simulink model "simulink_app"  (R2015a)
settings: Solver=ode2  SolverMode=SingleTasking  StartTime=0.0  StopTime=inf  FixedStep=T_ctrl  RelTol=1e-3
undefined symbols (not defined in the file): A_l_max_x, A_l_max_y, A_z_max, B_hover_4dof, CG_0, epsilon, eta_23, g, h, h_M, Hover_eta_23, Hover_throtle_1, Hover_throtle_23, I_BAC_0, Ix, Iy, Iz, l, l_arm, m, m_0, m_M, Rotation_sign, T_ctrl, throtle_1, throtle_23, v_i0
libraries: XXCopter_Control x52, simulink x11, XXCopter x1
(part 1 of 4)
settings Model: ExtModeTrigDuration=5000  Creator=DavidTorres  LastModifiedBy=David
settings SolverCC: AutoInsertRateTranBlk=on
settings DataIOCC: LimitDataPoints=off  SaveOutput=off  SignalLogging=off  DSMLogging=off  VisualizeSimOutput=off  SaveTime=off
settings OptimizationCC: InlineParams=on  UseFloatMulNetSlope=on  UseSpecifiedMinMax=on  InlineInvariantSignals=on  EnhancedBackFolding=on  PassReuseOutputArgsAs=Individual arguments  EfficientFloat2IntCast=on  EfficientMapNaN2IntZero=off  LifeSpan=Inf  MaxStackSize=64
settings DebuggingCC: WriteAfterWriteMsg=EnableAllAsError  SaveWithParameterizedLinksMsg=none  SignalResolutionControl=TryResolveAllWithWarning  IntegerOverflowMsg=error  ParameterUnderflowMsg=error  ParameterTunabilityLossMsg=error  UniqueDataStoreMsg=error  StrictBusMsg=ErrorOnBusTreatedAsVector  NonBusSignalsTreatedAsBus=error  SFUnexpectedBacktrackingDiag=error  SFInvalidInputDataAccessInChartInitDiag=error  SFNoUnconditionalDefaultTransitionDiag=error  SFTransitionOutsideNaturalParentDiag=error  SFUnconditionalTransitionShadowingDiag=error  SFUndirectedBroadcastEventsDiag=error  SFTransitionActionBeforeConditionDiag=error  IntegerSaturationMsg=error
settings HardwareCC: ProdLargestAtomicInteger=Long  ProdLargestAtomicFloat=Double  ProdEndianess=LittleEndian  ProdHWDeviceType=ARM Compatible->ARM Cortex
settings RTWCC: SystemTargetFile=ert.tlc  GenCodeOnly=on  TemplateMakefile=ert_default_tmf  Description=Embedded Coder  Toolchain=GNU Tools for ARM Embedded Processors  BuildConfiguration=Faster Runs
settings CodeAppCC: IgnoreCustomStorageClasses=off  IgnoreTestpoints=on
settings ERTTargetCC: UtilityFuncGeneration=Shared location  ParMdlRefBuildCompliant=on  CompOptLevelCompliant=on  ConcurrentExecutionCompliant=on  IncludeMdlTerminateFcn=off  ERTFirstTimeCompliant=on  ParenthesesLevel=Minimum  ModelStepFunctionPrototypeControlCompliant=on  CPPClassGenCompliant=on  ERTCustomFileTemplate=example_file_process.tlc  PreserveIfCondition=on  ConvertIfToSwitch=on

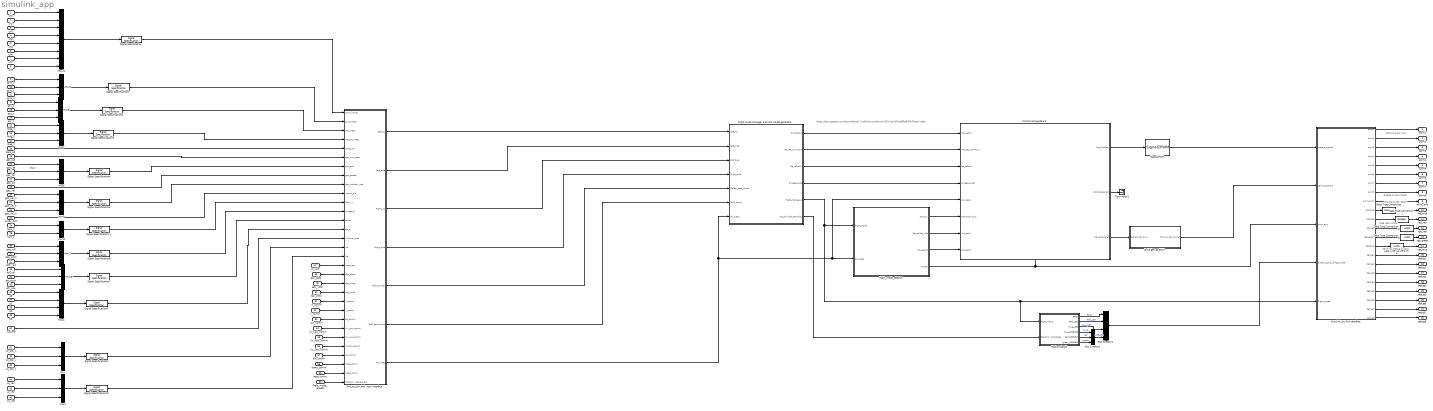
== system simulink_app ==
  note: degs!
  note: https://docs.google.com/document/d/17Lw5HdxcxpxePsmAYdCNVeyrDDt4j9EbtB6DkGHaHsY/edit
  note: Terminal Debug Output
  note: RGB LED (uint8)
  note: Standard LED (Bool)
  note: PWM Output (uS)
  note: Enable Output (Bool)
  ch1 : Inport  PortDimensions=[1,1]  SampleTime=T_ctrl
  ch2 : Inport  Port=2  PortDimensions=[1,1]  SampleTime=T_ctrl
  ch3 : Inport  Port=3  PortDimensions=[1,1]  SampleTime=T_ctrl
  ch4 : Inport  Port=4  PortDimensions=[1,1]  SampleTime=T_ctrl
  ch5 : Inport  Port=5  PortDimensions=[1,1]  SampleTime=T_ctrl
  ch6 : Inport  Port=6  PortDimensions=[1,1]  SampleTime=T_ctrl
  ch7 : Inport  Port=7  PortDimensions=[1,1]  SampleTime=T_ctrl
  ch8 : Inport  Port=8  PortDimensions=[1,1]  SampleTime=T_ctrl
  gyro_x : Inport  Port=9  PortDimensions=[1,1]  SampleTime=T_ctrl
  gyro_y : Inport  Port=10  PortDimensions=[1,1]  SampleTime=T_ctrl
  gyro_z : Inport  Port=11  PortDimensions=[1,1]  SampleTime=T_ctrl
  acc_x : Inport  Port=12  PortDimensions=[1,1]  SampleTime=T_ctrl
  acc_y : Inport  Port=13  PortDimensions=[1,1]  SampleTime=T_ctrl
  acc_z : Inport  Port=14  PortDimensions=[1,1]  SampleTime=T_ctrl
  mag_x : Inport  Port=15  PortDimensions=[1,1]  SampleTime=T_ctrl
  mag_y : Inport  Port=16  PortDimensions=[1,1]  SampleTime=T_ctrl
  mag_z : Inport  Port=17  PortDimensions=[1,1]  SampleTime=T_ctrl
  baro_alt : Inport  Port=18  PortDimensions=[1,1]  SampleTime=T_ctrl
  gps_sat : Inport  Port=19  PortDimensions=[1,1]  SampleTime=T_ctrl
  gps_lat : Inport  Port=20  PortDimensions=[1,1]  SampleTime=T_ctrl
  gps_lon : Inport  Port=21  PortDimensions=[1,1]  SampleTime=T_ctrl
  gps_alt : Inport  Port=22  PortDimensions=[1,1]  SampleTime=T_ctrl
  gps_vel : Inport  Port=23  PortDimensions=[1,1]  SampleTime=T_ctrl
  gps_vel_n : Inport  Port=24  PortDimensions=[1,1]  SampleTime=T_ctrl
  gps_vel_e : Inport  Port=25  PortDimensions=[1,1]  SampleTime=T_ctrl
  gps_vel_d : Inport  Port=26  PortDimensions=[1,1]  SampleTime=T_ctrl
  sonar_dist : Inport  Port=27  PortDimensions=[1,1]  SampleTime=T_ctrl
  flow_x : Inport  Port=28  PortDimensions=[1,1]  SampleTime=T_ctrl
  flow_y : Inport  Port=29  PortDimensions=[1,1]  SampleTime=T_ctrl
  rate_roll : Inport  Port=30  PortDimensions=[1,1]  SampleTime=T_ctrl
  rate_pitch : Inport  Port=31  PortDimensions=[1,1]  SampleTime=T_ctrl
  rate_yaw : Inport  Port=32  PortDimensions=[1,1]  SampleTime=T_ctrl
  att_roll : Inport  Port=33  PortDimensions=[1,1]  SampleTime=T_ctrl
  att_pitch : Inport  Port=34  PortDimensions=[1,1]  SampleTime=T_ctrl
  att_yaw : Inport  Port=35  PortDimensions=[1,1]  SampleTime=T_ctrl
  q0 : Inport  Port=36  PortDimensions=[1,1]  SampleTime=T_ctrl
  q1 : Inport  Port=37  PortDimensions=[1,1]  SampleTime=T_ctrl
  q2 : Inport  Port=38  PortDimensions=[1,1]  SampleTime=T_ctrl
  q3 : Inport  Port=39  PortDimensions=[1,1]  SampleTime=T_ctrl
  runtime : Inport  Port=40  PortDimensions=[1,1]  SampleTime=T_ctrl
  Lo_pos_x : Inport  Port=41  PortDimensions=[1,1]  SampleTime=T_ctrl
  Lo_pos_y : Inport  Port=42  PortDimensions=[1,1]  SampleTime=T_ctrl
  Lo_pos_z : Inport  Port=43  PortDimensions=[1,1]  SampleTime=T_ctrl
  Lo_vex : Inport  Port=44  PortDimensions=[1,1]  SampleTime=T_ctrl
  Lo_vey : Inport  Port=45  PortDimensions=[1,1]  SampleTime=T_ctrl
  Lo_vez : Inport  Port=46  PortDimensions=[1,1]  SampleTime=T_ctrl
  Lo_yaw : Inport  Port=47  PortDimensions=[1,1]  SampleTime=T_ctrl
  gps_pdop : Inport  Port=48  PortDimensions=[1,1]  SampleTime=T_ctrl
  gps_vdop : Inport  Port=49  PortDimensions=[1,1]  SampleTime=T_ctrl
  bat_volts : Inport  Port=50  PortDimensions=[1,1]  SampleTime=T_ctrl
  X_comm : Inport  Port=51  PortDimensions=[1,1]  SampleTime=T_ctrl
  Y_comm : Inport  Port=52  PortDimensions=[1,1]  SampleTime=T_ctrl
  Alt_comm : Inport  Port=53  PortDimensions=[1,1]  SampleTime=T_ctrl
  Vx_yaw_comm : Inport  Port=54  PortDimensions=[1,1]  SampleTime=T_ctrl
  Vy_yaw_comm : Inport  Port=55  PortDimensions=[1,1]  SampleTime=T_ctrl
  Vz_yaw_comm : Inport  Port=56  PortDimensions=[1,1]  SampleTime=T_ctrl
  phi_comm : Inport  Port=57  PortDimensions=[1,1]  SampleTime=T_ctrl
  theta_comm : Inport  Port=58  PortDimensions=[1,1]  SampleTime=T_ctrl
  head_comm : Inport  Port=59  PortDimensions=[1,1]  SampleTime=T_ctrl
  flight_mode_request : Inport  Port=60  PortDimensions=[1,1]  SampleTime=T_ctrl
  Build Servos PWM : Subsystem  TreatAsAtomicUnit=on
  Bus Creator1 : BusCreator
  Bus Creator2 : BusCreator  Inputs=3
  Control and guidance : Subsystem
  Data Type Conversion : DataTypeConversion  OutDataTypeStr=boolean
  Data Type Conversion1 : DataTypeConversion  OutDataTypeStr=boolean
  Data Type Conversion2 : DataTypeConversion  OutDataTypeStr=uint8
  Data Type Conversion3 : DataTypeConversion  OutDataTypeStr=uint8
  Data Type Conversion4 : DataTypeConversion  OutDataTypeStr=uint8
  Flight mode manager and commands generator : Subsystem
  Mux{,1..3,5..9} (9 alike) : Mux  Inputs=3
  Mux10 : Mux  Inputs=2
  Mux11 : Mux  Inputs=8
  Mux4 : Mux
  Px4_to_simulink input interface : Subsystem
  Signal Specification : SignalSpecification  Dimensions=[8,1]
  Signal Specification{1..7,9..10} (9 alike) : SignalSpecification  Dimensions=[3,1]
  Signal Specification11 : SignalSpecification  Dimensions=[2,1]
  Signal Specification8 : SignalSpecification  Dimensions=[4,1]
  Signal2PWM : XXCopter_Control/Signal2PWM  b=1  d=0  a=1800  c=1200
  Simulink_to_Px4 interface : Subsystem
  Status signals : Subsystem  TreatAsAtomicUnit=on
  Terminator1 : Terminator
  flight_mode_effector : Subsystem
  pwm1 : Outport  PortDimensions=[1,1]
  pwm2 : Outport  Port=2  PortDimensions=[1,1]
  pwm3 : Outport  Port=3  PortDimensions=[1,1]
  pwm4 : Outport  Port=4  PortDimensions=[1,1]
  pwm5 : Outport  Port=5  PortDimensions=[1,1]
  pwm6 : Outport  Port=6  PortDimensions=[1,1]
  pwm7 : Outport  Port=7  PortDimensions=[1,1]
  pwm8 : Outport  Port=8  PortDimensions=[1,1]
  pwm_arm : Outport  Port=9  PortDimensions=[1,1]
  led_blue : Outport  Port=10  OutDataTypeStr=boolean  PortDimensions=[1,1]
  led_red : Outport  Port=11  OutDataTypeStr=boolean  PortDimensions=[1,1]
  rgb_red : Outport  Port=12  OutDataTypeStr=uint8  PortDimensions=[1,1]
  rgb_green : Outport  Port=13  OutDataTypeStr=uint8  PortDimensions=[1,1]
  rgb_blue : Outport  Port=14  OutDataTypeStr=uint8  PortDimensions=[1,1]
  debug1 : Outport  Port=15  PortDimensions=[1,1]
  debug2 : Outport  Port=16  PortDimensions=[1,1]
  debug3 : Outport  Port=17  PortDimensions=[1,1]
  debug4 : Outport  Port=18  PortDimensions=[1,1]
  debug5 : Outport  Port=19  PortDimensions=[1,1]
  debug6 : Outport  Port=20  PortDimensions=[1,1]
  debug7 : Outport  Port=21  PortDimensions=[1,1]
  debug8 : Outport  Port=22  PortDimensions=[1,1]
  wires:
  Flight mode manager and commands generator/1(Pos_ref(m)) -> Control and guidance/1(Pos_ref(m))
  Flight mode manager and commands generator/2(Vel_ref_yaw(mps)) -> Control and guidance/2(Vel_ref_yaw(mps))
  Flight mode manager and commands generator/3(Att_ref(rad)) -> Control and guidance/3(Att_ref(rad))
  Control and guidance/1(Mot_throtles) -> Signal2PWM/1
  Control and guidance/3(Servos_angles) -> Build Servos PWM/1(signals servos in)
  Flight mode manager and commands generator/4(omega_b_ref) -> Control and guidance/4(omega_b_ref)
  flight_mode_effector/1(Act_bus) -> Control and guidance/6(activation_bus)
  flight_mode_effector/2(Controller_inits) -> Control and guidance/7(Init_cond)
  flight_mode_effector/3(CA_reconf) -> Control and guidance/8(CA_reconf)
  Flight mode manager and commands generator/6(not_allowed_transition) -> Status signals/2(Not_allowed_change)
  Status signals/1(Beep) -> Bus Creator1/1  "Beep"
  Status signals/2(Red_LED) -> Bus Creator1/2  "Red_LED"
  Status signals/3(blue_LED) -> Bus Creator1/3  "blue_LED"
  Status signals/4(blue_RGBLED) -> Bus Creator2/1  "blue"
  Status signals/5(Red_RGBLED) -> Bus Creator2/2  "red"
  Status signals/6(green_RGBLED) -> Bus Creator2/3  "green"
  Bus Creator2/1 -> Bus Creator1/4  "RGBLED"
  Simulink_to_Px4 interface/1(pwm1) -> pwm1/1
  Simulink_to_Px4 interface/2(pwm2) -> pwm2/1
  Simulink_to_Px4 interface/3(pwm3) -> pwm3/1
  Simulink_to_Px4 interface/4(pwm4) -> pwm4/1
  Simulink_to_Px4 interface/5(pwm5) -> pwm5/1
  Simulink_to_Px4 interface/6(pwm6) -> pwm6/1
  Simulink_to_Px4 interface/7(pwm7) -> pwm7/1
  Simulink_to_Px4 interface/8(pwm8) -> pwm8/1
  Simulink_to_Px4 interface/10(led_blue) -> Data Type Conversion/1
  Simulink_to_Px4 interface/11(led_red) -> Data Type Conversion1/1
  Simulink_to_Px4 interface/15(debug1) -> debug1/1
  Simulink_to_Px4 interface/17(debug3) -> debug3/1
  Simulink_to_Px4 interface/18(debug4) -> debug4/1
  Simulink_to_Px4 interface/9(pwm_arm1) -> pwm_arm/1
  Simulink_to_Px4 interface/12(rgb_red) -> Data Type Conversion2/1
  Simulink_to_Px4 interface/13(rgb_green) -> Data Type Conversion3/1
  Simulink_to_Px4 interface/14(rgb_blue) -> Data Type Conversion4/1
  Simulink_to_Px4 interface/20(debug6) -> debug6/1
  Simulink_to_Px4 interface/21(debug7) -> debug7/1
  Simulink_to_Px4 interface/22(debug8) -> debug8/1
  Simulink_to_Px4 interface/19(debug5) -> debug5/1
  flight_mode_effector/4(Armed) -> Simulink_to_Px4 interface/3(pwm_arm), Control and guidance/Enable
  Data Type Conversion/1 -> led_blue/1
  Data Type Conversion1/1 -> led_red/1
  Flight mode manager and commands generator/5(flight_mode_out) -> Simulink_to_Px4 interface/5(flight_mode), Status signals/1(flight_mode), flight_mode_effector/1(flight_mode)
  Data Type Conversion2/1 -> rgb_red/1
  Data Type Conversion3/1 -> rgb_green/1
  Data Type Conversion4/1 -> rgb_blue/1
  Control and guidance/2(Control_signals) -> Terminator1/1
  Simulink_to_Px4 interface/16(debug2) -> debug2/1
  Signal2PWM/1 -> Simulink_to_Px4 interface/1(motors_signals)
  Build Servos PWM/1(PWM_us servos out) -> Simulink_to_Px4 interface/2(servos_signals)
  Bus Creator1/1 -> Simulink_to_Px4 interface/4(extern_signal_flihgt_mode)
  Px4_to_simulink input interface/7(All_meas) -> Control and guidance/5(All_meas), flight_mode_effector/2(All_meas), Flight mode manager and commands generator/7(All_meas)
  sonar_dist/1 -> Px4_to_simulink input interface/10(usonic_alt)
  baro_alt/1 -> Px4_to_simulink input interface/5(press_alt)
  gyro_z/1 -> Mux6/3
  gyro_y/1 -> Mux6/2
  gyro_x/1 -> Mux6/1
  acc_z/1 -> Mux5/3
  acc_y/1 -> Mux5/2
  acc_x/1 -> Mux5/1
  mag_x/1 -> Mux7/1
  mag_y/1 -> Mux7/2
  mag_z/1 -> Mux7/3
  ch1/1 -> Mux11/1
  ch2/1 -> Mux11/2
  ch3/1 -> Mux11/3
  ch4/1 -> Mux11/4
  ch5/1 -> Mux11/5
  ch6/1 -> Mux11/6
  flow_y/1 -> Mux10/2
  flow_x/1 -> Mux10/1
  runtime/1 -> Px4_to_simulink input interface/15(runtime_usec)
  ch7/1 -> Mux11/7
  ch8/1 -> Mux11/8
  att_roll/1 -> Mux3/1
  att_pitch/1 -> Mux3/2
  att_yaw/1 -> Mux3/3
  q0/1 -> Mux4/1
  q1/1 -> Mux4/2
  q2/1 -> Mux4/3
  q3/1 -> Mux4/4
  rate_roll/1 -> Mux2/1
  rate_pitch/1 -> Mux2/2
  rate_yaw/1 -> Mux2/3
  gps_vel_n/1 -> Mux9/1
  gps_vel_e/1 -> Mux9/2
  gps_vel_d/1 -> Mux9/3
  gps_lat/1 -> Mux8/1
  gps_lon/1 -> Mux8/2
  gps_alt/1 -> Mux8/3
  gps_vel/1 -> Px4_to_simulink input interface/8(gps_speed)
  gps_sat/1 -> Px4_to_simulink input interface/6(gps_num_sats)
  Lo_pos_x/1 -> Mux/1
  Lo_pos_y/1 -> Mux/2
  Lo_pos_z/1 -> Mux/3
  Mux/1 -> Signal Specification9/1
  Lo_vex/1 -> Mux1/1
  Lo_vey/1 -> Mux1/2
  Lo_vez/1 -> Mux1/3
  Mux1/1 -> Signal Specification10/1
  Mux2/1 -> Signal Specification6/1
  Mux3/1 -> Signal Specification7/1
  Mux4/1 -> Signal Specification8/1
  Mux5/1 -> Signal Specification2/1
  Y_comm/1 -> Px4_to_simulink input interface/23(Y_comm)
  Alt_comm/1 -> Px4_to_simulink input interface/24(Alt_comm)
  Vx_yaw_comm/1 -> Px4_to_simulink input interface/25(Vx_yaw_comm)
  Vy_yaw_comm/1 -> Px4_to_simulink input interface/26(Vy_yaw_comm)
  theta_comm/1 -> Px4_to_simulink input interface/29(theta_comm)
  head_comm/1 -> Px4_to_simulink input interface/30(head_comm)
  flight_mode_request/1 -> Px4_to_simulink input interface/31(flight_mode_request)
  Mux6/1 -> Signal Specification1/1
  Mux8/1 -> Signal Specification4/1
  Mux7/1 -> Signal Specification3/1
  Mux11/1 -> Signal Specification/1
  Mux10/1 -> Signal Specification11/1
  Mux9/1 -> Signal Specification5/1
  Lo_yaw/1 -> Px4_to_simulink input interface/18(Local_taw)
  gps_pdop/1 -> Px4_to_simulink input interface/19(gps_pdop)
  gps_vdop/1 -> Px4_to_simulink input interface/20(gps_vdop)
  bat_volts/1 -> Px4_to_simulink input interface/21(bat_volts)
  X_comm/1 -> Px4_to_simulink input interface/22(X_comm)
  Vz_yaw_comm/1 -> Px4_to_simulink input interface/27(Vz_yaw_comm)
  phi_comm/1 -> Px4_to_simulink input interface/28(phi_comm)
  Px4_to_simulink input interface/1(Left_up) -> Flight mode manager and commands generator/1(Left_up)
  Px4_to_simulink input interface/2(Left_side) -> Flight mode manager and commands generator/2(Left_side)
  Px4_to_simulink input interface/3(Right_up) -> Flight mode manager and commands generator/3(Right_up)
  Px4_to_simulink input interface/4(Right_side) -> Flight mode manager and commands generator/4(Right_side)
  Px4_to_simulink input interface/5(radio_siwtch) -> Flight mode manager and commands generator/5(Safety_stab_switch)
  Px4_to_simulink input interface/6(GCS_commands) -> Flight mode manager and commands generator/6(GCS_comm)
  Signal Specification/1 -> Px4_to_simulink input interface/1(pwm_inputs)
  Signal Specification1/1 -> Px4_to_simulink input interface/2(gyro_meas)
  Signal Specification2/1 -> Px4_to_simulink input interface/3(acc_meas)
  Signal Specification3/1 -> Px4_to_simulink input interface/4(magne_meas)
  Signal Specification4/1 -> Px4_to_simulink input interface/7(gps_pos)
  Signal Specification5/1 -> Px4_to_simulink input interface/9(gps_velocity_ned)
  Signal Specification6/1 -> Px4_to_simulink input interface/12(omega_b)
  Signal Specification7/1 -> Px4_to_simulink input interface/13(euler)
  Signal Specification8/1 -> Px4_to_simulink input interface/14(att_q)
  Signal Specification9/1 -> Px4_to_simulink input interface/16(Xe)
  Signal Specification10/1 -> Px4_to_simulink input interface/17(Ve)
  Signal Specification11/1 -> Px4_to_simulink input interface/11(flow_xy)

== system simulink_app/Build Servos PWM ==
  note: Control input
      | Rango
      | Direccion rot/Dir servos
      | Rango del servo
      |
      | eta_1 (rad) (Pan arm 1)
      | -165,165
      | -1
      | 330: -165,165
      |
      | gamma_1 (rad) (Tilt arm 1)
      | -90,15
      | -1
      | 180:-90,90 ó 330: -165,165
      |
      | eta_2 (rad) (Pan arm 2)
      | -165,165
      | -1
      | 330: -165,165
      |
      | gamma_2 (rad) (Tilt arm 2)
      | -15,90
      | 1
      | 180:-90,90
      |
      | eta_3 (rad) (Pan arm 3)
      | -165,165
      | 1
      | 330:-165,165
      |
      | gamma_3 (rad) (Tilt arm 3)
      | -90,15
      | -1
      | 180:-90,90
  signals servos in : Inport
  Demux : Demux  Outputs=6
  Mux : Mux  Inputs=6
  Signal2PWM1 : XXCopter_Control/Signal2PWM  b=deg2rad(165)  d=-deg2rad(165)  a=2100  c=900
  Signal2PWM2 : XXCopter_Control/Signal2PWM  b=deg2rad(90)  d=-deg2rad(90)  a=2100  c=900
  Signal2PWM3 : XXCopter_Control/Signal2PWM  b=deg2rad(90)  d=-deg2rad(90)  a=2100  c=900
  Signal2PWM4 : XXCopter_Control/Signal2PWM  b=deg2rad(90)  d=-deg2rad(90)  a=2100  c=900
  Signal2PWM5 : XXCopter_Control/Signal2PWM  b=deg2rad(165)  d=-deg2rad(165)  a=2100  c=900
  Signal2PWM6 : XXCopter_Control/Signal2PWM  b=deg2rad(165)  d=-deg2rad(165)  a=2100  c=900
  Unary Minus{,1..3} (4 alike) : UnaryMinus
  PWM_us servos out : Outport
  wires:
  signals servos in/1 -> Demux/1
  Demux/1 -> Unary Minus/1
  Demux/2 -> Unary Minus1/1
  Demux/3 -> Unary Minus2/1
  Demux/6 -> Unary Minus3/1
  Unary Minus3/1 -> Signal2PWM3/1
  Demux/5 -> Signal2PWM6/1
  Demux/4 -> Signal2PWM4/1
  Unary Minus2/1 -> Signal2PWM5/1
  Unary Minus1/1 -> Signal2PWM2/1
  Unary Minus/1 -> Signal2PWM1/1
  Signal2PWM1/1 -> Mux/1
  Signal2PWM2/1 -> Mux/2
  Signal2PWM5/1 -> Mux/3
  Signal2PWM4/1 -> Mux/4
  Signal2PWM6/1 -> Mux/5
  Signal2PWM3/1 -> Mux/6
  Mux/1 -> PWM_us servos out/1

== system simulink_app/Control and guidance ==
  Pos_ref(m) : Inport
  Vel_ref_yaw(mps) : Inport  Port=2
  Att_ref(rad) : Inport  Port=3
  omega_b_ref : Inport  Port=4
  All_meas : Inport  Port=5
  activation_bus : Inport  Port=6
  Init_cond : Inport  Port=7
  CA_reconf : Inport  Port=8
  Enable : EnablePort  StatesWhenEnabling=reset
  Bus Selector : BusSelector  OutputSignals=Meas.Volt
  Control allocator : Subsystem  RTWFcnName=abc  RTWFileName=asas  VariantControl=Control Allocator: NO RECONFIG
      settings: MinAlgLoopOccurrences=on  RTWFcnNameOpts=User specified  RTWFileNameOpts=User specified
  Demux : Demux  Outputs=3
  Equivalent ESC signals : Product  Inputs=/*
  Equivalent Throttle : Product  Inputs=**
  Initial control deflections : Memory  X0=[throtle_1,0,0,throtle_23,eta_23,0,throtle_23,-eta_23,0]'  InheritSampleTime=on
  Inner PI Controller Quaternions : Subsystem  VariantControl=PI_quat
  NDI : Subsystem  RTWFcnName=abc  RTWFileName=asas  VariantControl=NDI: NO RECONFIG
      settings: RTWFcnNameOpts=User specified  RTWFileNameOpts=User specified
  Otter Overactuated P Controller : Subsystem  VariantControl=Overactuated P Controller
  Reference batrery level (V) : Constant  Value=16
  Safety limits : Saturate  UpperLimit=[20,20,0]'  LowerLimit=-[20,20,50]'
  Saturation1 : Saturate  UpperLimit=[10,10,v_i0]'  LowerLimit=-[10,10,2*v_i0]'
  Throttles : Selector  InputPortWidth=9  Indices=[1,4,7]
  "angles " : Selector  InputPortWidth=9  Indices=[2,3,5,6,8,9]
  keep -90/90 : Subsystem
  Mot_throtles : Outport
  Control_signals : Outport  Port=2
  Servos_angles : Outport  Port=3
  wires:
  All_meas/1 -> Otter Overactuated P Controller/3(All meas), Inner PI Controller Quaternions/6(All meas), Bus Selector/1, NDI/3(All_meas)
  NDI/3(Control_defl eval (rad)) -> Control allocator/4(Control defl prev)
  keep -90/90/1(out (rad)) -> Demux/1
  Demux/3 -> Inner PI Controller Quaternions/4(Yaw_ref (rad))
  Demux/2 -> Inner PI Controller Quaternions/3(Theta_ref (rad))
  Demux/1 -> Inner PI Controller Quaternions/2(Phi_ref (rad))
  Otter Overactuated P Controller/1(Accels des) -> Inner PI Controller Quaternions/1(Accels ref (m/s^2))
  Safety limits/1 -> Otter Overactuated P Controller/1(Position ref (m))
  Att_ref(rad)/1 -> keep -90/90/1(in (rad))
  Equivalent Throttle/1 -> Equivalent ESC signals/2
  Reference batrery level (V)/1 -> Equivalent Throttle/1
  Bus Selector/1 -> Control allocator/1(Curr_V), Equivalent ESC signals/1  "<Volt>"
  Equivalent ESC signals/1 -> Mot_throtles/1
  Control allocator/1(Control_Commands) -> "angles "/1, Control_signals/1, Throttles/1
  Throttles/1 -> Equivalent Throttle/2
  Initial control deflections/1 -> NDI/2(Control_defl for eval)
  "angles "/1 -> Servos_angles/1
  Vel_ref_yaw(mps)/1 -> Saturation1/1
  Saturation1/1 -> Otter Overactuated P Controller/2(Vel_yaw_ref(m))
  Pos_ref(m)/1 -> Safety limits/1
  Init_cond/1 -> Otter Overactuated P Controller/5(init_cond), Inner PI Controller Quaternions/8(init_cond)
  CA_reconf/1 -> Control allocator/5(CA_reconf)
  activation_bus/1 -> Otter Overactuated P Controller/4(activation_bus), Inner PI Controller Quaternions/7(activation_bus)
  Control allocator/2(Control_def for eval) -> Initial control deflections/1
  NDI/1(Virtual Control Commands) -> Control allocator/2(Forc_Mom_des)
  NDI/2(B online) -> Control allocator/3(B matrix Online)
  Inner PI Controller Quaternions/1(Accs_Ang_acc des) -> NDI/1(pseudo_control (m/s^2;rad/s^2))
  omega_b_ref/1 -> Inner PI Controller Quaternions/5(omega_b_ref_radps)

== system simulink_app/Flight mode manager and commands generator ==
  Left_up : Inport
  Left_side : Inport  Port=2
  Right_up : Inport  Port=3
  Right_side : Inport  Port=4
  Safety_stab_switch : Inport  Port=5
  GCS_comm : Inport  Port=6
  All_meas : Inport  Port=7
  Bus Selector : BusSelector  OutputSignals=flight_mode_request
  Commands generator : Subsystem
  Flight manager : Subsystem
  Pos_ref(m) : Outport  PortDimensions=[3,1]
  Vel_ref_yaw(mps) : Outport  Port=2  PortDimensions=[3,1]
  Att_ref(rad) : Outport  Port=3  PortDimensions=[3,1]
  omega_b_ref : Outport  Port=4  PortDimensions=[3,1]
  flight_mode_out : Outport  Port=5
  not_allowed_transition : Outport  Port=6
  wires:
  Flight manager/1(flight_mode) -> Commands generator/1(flight_mode), flight_mode_out/1
  All_meas/1 -> Flight manager/2(All_meas), Commands generator/7(All_meas)
  Commands generator/1(Pos_ref(m)) -> Pos_ref(m)/1
  Commands generator/3(Att_ref(rad)) -> Att_ref(rad)/1
  Commands generator/2(Vel_ref_yaw(mps)) -> Vel_ref_yaw(mps)/1
  Commands generator/4(omega_b_ref) -> omega_b_ref/1
  GCS_comm/1 -> Bus Selector/1, Commands generator/6(GCS_comm)
  Bus Selector/1 -> Flight manager/1(flight_mode_request)  "<flight_mode_request>"
  Safety_stab_switch/1 -> Flight manager/3(Safety_stab_switch)
  Left_up/1 -> Commands generator/2(Left_up)
  Left_side/1 -> Commands generator/3(Left_side)
  Right_up/1 -> Commands generator/4(Right_up)
  Right_side/1 -> Commands generator/5(Right_side)
  Flight manager/2(not_allowed_transition) -> not_allowed_transition/1

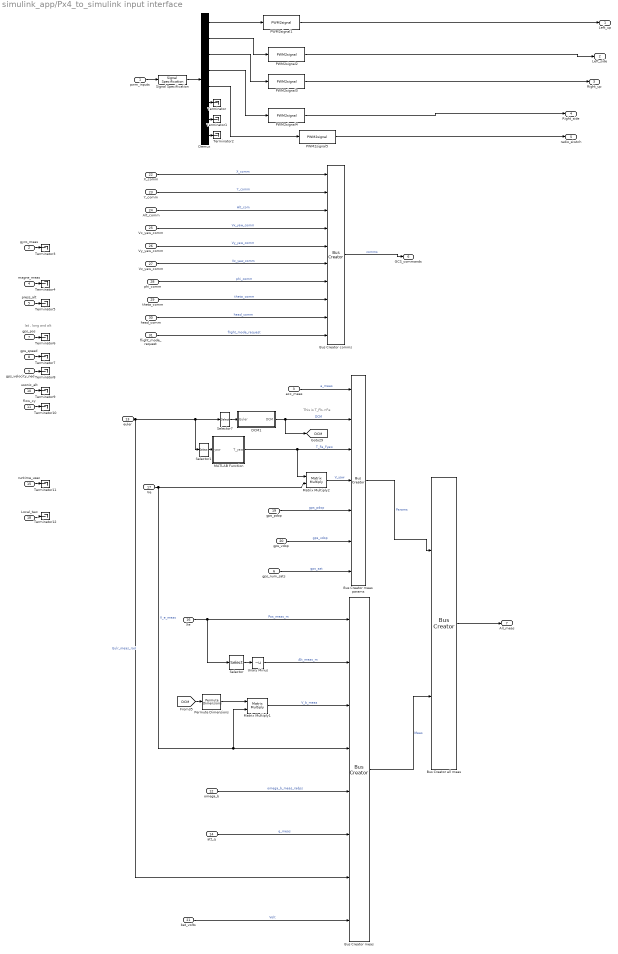
== system simulink_app/Px4_to_simulink input interface ==
  note: lat , long and alt
  note: This is T_Fb->Fe
  pwm_inputs : Inport  PortDimensions=8  SampleTime=T_ctrl
  gyro_meas : Inport  Port=2  PortDimensions=3  SampleTime=T_ctrl
  acc_meas : Inport  Port=3  PortDimensions=3  SampleTime=T_ctrl
  magne_meas : Inport  Port=4  PortDimensions=3  SampleTime=T_ctrl
  press_alt : Inport  Port=5  PortDimensions=1  SampleTime=T_ctrl
  gps_num_sats : Inport  Port=6  PortDimensions=1  SampleTime=T_ctrl
  gps_pos : Inport  Port=7  PortDimensions=3  SampleTime=T_ctrl
  gps_speed : Inport  Port=8  PortDimensions=1  SampleTime=T_ctrl
  gps_velocity_ned : Inport  Port=9  PortDimensions=3  SampleTime=T_ctrl
  usonic_alt : Inport  Port=10  PortDimensions=1  SampleTime=T_ctrl
  flow_xy : Inport  Port=11  PortDimensions=2  SampleTime=T_ctrl
  omega_b : Inport  Port=12  PortDimensions=3  SampleTime=T_ctrl
  euler : Inport  Port=13  PortDimensions=3  SampleTime=T_ctrl
  att_q : Inport  Port=14  PortDimensions=4  SampleTime=T_ctrl
  runtime_usec : Inport  Port=15  PortDimensions=1  SampleTime=T_ctrl
  Xe : Inport  Port=16  PortDimensions=3  SampleTime=T_ctrl
  Ve : Inport  Port=17  PortDimensions=3  SampleTime=T_ctrl
  Local_taw : Inport  Port=18  PortDimensions=1  SampleTime=T_ctrl
  gps_pdop : Inport  Port=19  PortDimensions=1  SampleTime=T_ctrl
  gps_vdop : Inport  Port=20  PortDimensions=1  SampleTime=T_ctrl
  bat_volts : Inport  Port=21  PortDimensions=1  SampleTime=T_ctrl
  X_comm : Inport  Port=22  PortDimensions=1  SampleTime=T_ctrl
  Y_comm : Inport  Port=23  PortDimensions=1  SampleTime=T_ctrl
  Alt_comm : Inport  Port=24  PortDimensions=1  SampleTime=T_ctrl
  Vx_yaw_comm : Inport  Port=25  PortDimensions=[1,1]
  Vy_yaw_comm : Inport  Port=26  PortDimensions=1  SampleTime=T_ctrl
  Vz_yaw_comm : Inport  Port=27  PortDimensions=1  SampleTime=T_ctrl
  phi_comm : Inport  Port=28  PortDimensions=1  SampleTime=T_ctrl
  theta_comm : Inport  Port=29  PortDimensions=1  SampleTime=T_ctrl
  head_comm : Inport  Port=30  PortDimensions=1  SampleTime=T_ctrl
  flight_mode_request : Inport  Port=31  PortDimensions=1  SampleTime=T_ctrl
  Bus Creator all meas : BusCreator  Inputs=2  OutDataTypeStr=Bus: slBus2
  Bus Creator comms : BusCreator  Inputs=10  OutDataTypeStr=Bus: slBus1_comms
  Bus Creator meas : BusCreator  Inputs=8  OutDataTypeStr=Bus: Meas
  Bus Creator meas params : BusCreator  Inputs=7  OutDataTypeStr=Bus: Params
  DCM1 : Subsystem  TreatAsAtomicUnit=on
  Demux : Demux  Outputs=8
  MATLAB Function : MATLAB Function  TreatAsAtomicUnit=on
  Matrix Multiply1 : Product  Multiplication=Matrix(*)
  Matrix Multiply2 : Product  Multiplication=Matrix(*)
  PWM2signal{1..4} (4 alike) : XXCopter_Control/PWM2signal  c=1800  a=1200  d=1  b=-1
  PWM2signal5 : XXCopter_Control/PWM2signal  c=1800  a=1200  d=1  b=0
  Permute Dimensions : PermuteDimensions
  Selector : Selector  InputPortWidth=3  Indices=3
  Selector1 : Selector  InputPortWidth=3  Indices=3
  Selector7 : Selector  InputPortWidth=3  Indices=[3 2 1]
  Signal Specification : SignalSpecification  Dimensions=8
  Terminator{,1..12} (13 alike) : Terminator
  Unary Minus : UnaryMinus
  Left_up : Outport
  Left_side : Outport  Port=2
  Right_up : Outport  Port=3
  Right_side : Outport  Port=4
  radio_siwtch : Outport  Port=5
  GCS_commands : Outport  Port=6
  All_meas : Outport  Port=7
  tag scope: DCM=global
  wires:
  PWM2signal1/1 -> Left_up/1
  PWM2signal2/1 -> Left_side/1
  PWM2signal3/1 -> Right_up/1
  PWM2signal4/1 -> Right_side/1
  Bus Creator all meas/1 -> All_meas/1
  PWM2signal5/1 -> radio_siwtch/1
  Xe/1 -> Selector/1, Bus Creator meas/1  "Pos_meas_m"
  att_q/1 -> Bus Creator meas/6  "q_meas"
  Ve/1 -> Bus Creator meas/4, Matrix Multiply1/2, Matrix Multiply2/2  "V_e_meas"
  euler/1 -> Bus Creator meas/7, Selector1/1, Selector7/1  "Eulr_meas_rad"
  omega_b/1 -> Bus Creator meas/5  "omega_b_meas_radps"
  Matrix Multiply1/1 -> Bus Creator meas/3  "V_b_meas"
  Unary Minus/1 -> Bus Creator meas/2  "Alt_meas_m"
  Selector/1 -> Unary Minus/1
  bat_volts/1 -> Bus Creator meas/8  "Volt"
  Bus Creator meas/1 -> Bus Creator all meas/2  "Meas"
  Bus Creator meas params/1 -> Bus Creator all meas/1  "Params"
  DCM1/1(DCM) -> [DCM], Bus Creator meas params/2  "DCM"
  Matrix Multiply2/1 -> Bus Creator meas params/4  "V_yaw"
  acc_meas/1 -> Bus Creator meas params/1  "a_meas"
  gps_pdop/1 -> Bus Creator meas params/5  "gps_pdop"
  gps_num_sats/1 -> Bus Creator meas params/7  "gps_sat"
  gps_vdop/1 -> Bus Creator meas params/6  "gps_vdop"
  Selector7/1 -> DCM1/1(Euler)
  Selector1/1 -> MATLAB Function/1(yaw)
  MATLAB Function/1(T_yaw) -> Matrix Multiply2/1, Bus Creator meas params/3  "T_Fe_Fyaw"
  [DCM] -> Permute Dimensions/1
  Permute Dimensions/1 -> Matrix Multiply1/1
  Bus Creator comms/1 -> GCS_commands/1  "comms"
  X_comm/1 -> Bus Creator comms/1  "X_comm"
  flight_mode_request/1 -> Bus Creator comms/10  "flight_mode_request"
  Y_comm/1 -> Bus Creator comms/2  "Y_comm"
  Vx_yaw_comm/1 -> Bus Creator comms/4  "Vx_yaw_comm"
  Vy_yaw_comm/1 -> Bus Creator comms/5  "Vy_yaw_comm"
  Vz_yaw_comm/1 -> Bus Creator comms/6  "Vz_yaw_comm"
  phi_comm/1 -> Bus Creator comms/7  "phi_comm"
  theta_comm/1 -> Bus Creator comms/8  "theta_comm"
  head_comm/1 -> Bus Creator comms/9  "head_comm"
  Demux/1 -> PWM2signal1/1
  Demux/2 -> PWM2signal2/1
  Demux/3 -> PWM2signal3/1
  Demux/4 -> PWM2signal4/1
  Demux/5 -> PWM2signal5/1
  Alt_comm/1 -> Bus Creator comms/3  "Alt_com"
  pwm_inputs/1 -> Signal Specification/1
  Demux/6 -> Terminator/1
  Demux/7 -> Terminator1/1
  Demux/8 -> Terminator2/1
  gyro_meas/1 -> Terminator3/1
  magne_meas/1 -> Terminator4/1
  press_alt/1 -> Terminator5/1
  gps_pos/1 -> Terminator6/1
  gps_speed/1 -> Terminator7/1
  gps_velocity_ned/1 -> Terminator8/1
  usonic_alt/1 -> Terminator9/1
  flow_xy/1 -> Terminator10/1
  runtime_usec/1 -> Terminator11/1
  Local_taw/1 -> Terminator12/1
  Signal Specification/1 -> Demux/1

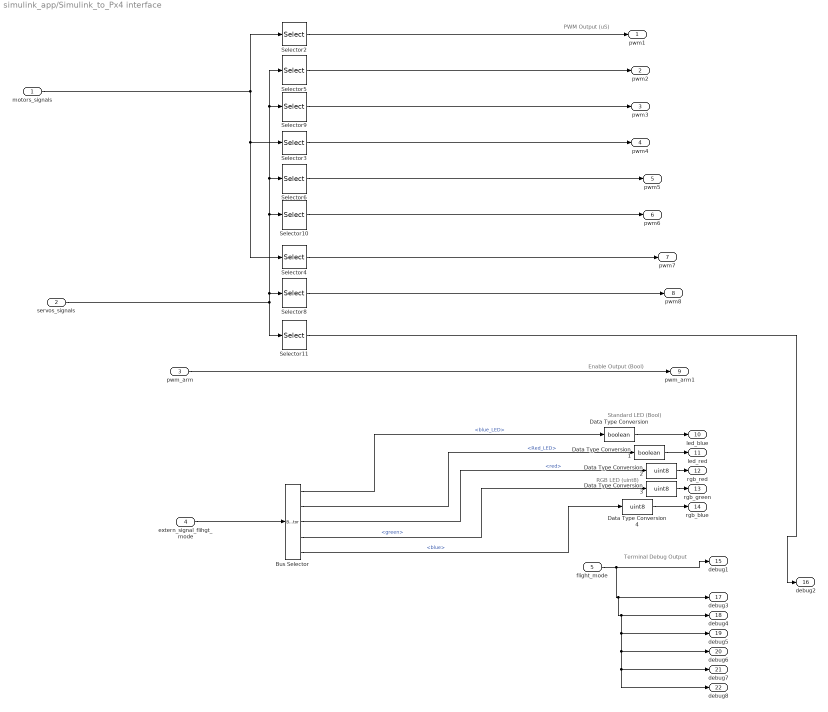
== system simulink_app/Simulink_to_Px4 interface ==
  note: Terminal Debug Output
  note: RGB LED (uint8)
  note: Standard LED (Bool)
  note: PWM Output (uS)
  note: Enable Output (Bool)
  motors_signals : Inport
  servos_signals : Inport  Port=2
  pwm_arm : Inport  Port=3
  extern_signal_flihgt_mode : Inport  Port=4
  flight_mode : Inport  Port=5
  Bus Selector : BusSelector  OutputSignals=blue_LED,Red_LED,RGBLED.red,RGBLED.green,RGBLED.blue
  Data Type Conversion : DataTypeConversion  OutDataTypeStr=boolean
  Data Type Conversion1 : DataTypeConversion  OutDataTypeStr=boolean
  Data Type Conversion2 : DataTypeConversion  OutDataTypeStr=uint8
  Data Type Conversion3 : DataTypeConversion  OutDataTypeStr=uint8
  Data Type Conversion4 : DataTypeConversion  OutDataTypeStr=uint8
  Selector10 : Selector  InputPortWidth=6  Indices=4
  Selector11 : Selector  InputPortWidth=6  Indices=6
  Selector2 : Selector  InputPortWidth=3
  Selector3 : Selector  InputPortWidth=3  Indices=2
  Selector4 : Selector  InputPortWidth=3  Indices=3
  Selector5 : Selector  InputPortWidth=6  Indices=[1]
  Selector6 : Selector  InputPortWidth=6  Indices=[3]
  Selector8 : Selector  InputPortWidth=6  Indices=5
  Selector9 : Selector  InputPortWidth=6  Indices=[2]
  pwm1 : Outport  PortDimensions=1  SampleTime=T_ctrl
  pwm2 : Outport  Port=2  PortDimensions=1  SampleTime=T_ctrl
  pwm3 : Outport  Port=3  PortDimensions=1  SampleTime=T_ctrl
  pwm4 : Outport  Port=4  PortDimensions=1  SampleTime=T_ctrl
  pwm5 : Outport  Port=5  PortDimensions=1  SampleTime=T_ctrl
  pwm6 : Outport  Port=6  PortDimensions=1  SampleTime=T_ctrl
  pwm7 : Outport  Port=7  PortDimensions=1  SampleTime=T_ctrl
  pwm8 : Outport  Port=8  PortDimensions=1  SampleTime=T_ctrl
  pwm_arm1 : Outport  Port=9  PortDimensions=1  SampleTime=T_ctrl
  led_blue : Outport  Port=10  OutDataTypeStr=boolean  PortDimensions=1  SampleTime=T_ctrl
  led_red : Outport  Port=11  OutDataTypeStr=boolean  PortDimensions=1  SampleTime=T_ctrl
  rgb_red : Outport  Port=12  OutDataTypeStr=uint8  PortDimensions=1  SampleTime=T_ctrl
  rgb_green : Outport  Port=13  OutDataTypeStr=uint8  PortDimensions=1  SampleTime=T_ctrl
  rgb_blue : Outport  Port=14  OutDataTypeStr=uint8  PortDimensions=1  SampleTime=T_ctrl
  debug1 : Outport  Port=15  PortDimensions=1  SampleTime=T_ctrl
  debug2 : Outport  Port=16  PortDimensions=1  SampleTime=T_ctrl
  debug3 : Outport  Port=17  PortDimensions=1  SampleTime=T_ctrl
  debug4 : Outport  Port=18  PortDimensions=1  SampleTime=T_ctrl
  debug5 : Outport  Port=19  PortDimensions=1  SampleTime=T_ctrl
  debug6 : Outport  Port=20  PortDimensions=1  SampleTime=T_ctrl
  debug7 : Outport  Port=21  PortDimensions=1  SampleTime=T_ctrl
  debug8 : Outport  Port=22  PortDimensions=1  SampleTime=T_ctrl
  wires:
  motors_signals/1 -> Selector3/1, Selector4/1, Selector2/1
  servos_signals/1 -> Selector9/1, Selector5/1, Selector6/1, Selector10/1, Selector8/1, Selector11/1
  extern_signal_flihgt_mode/1 -> Bus Selector/1
  Bus Selector/2 -> Data Type Conversion1/1  "<Red_LED>"
  Selector2/1 -> pwm1/1
  Selector5/1 -> pwm2/1
  Selector9/1 -> pwm3/1
  Selector3/1 -> pwm4/1
  Selector6/1 -> pwm5/1
  Selector10/1 -> pwm6/1
  Selector4/1 -> pwm7/1
  Selector8/1 -> pwm8/1
  pwm_arm/1 -> pwm_arm1/1
  Bus Selector/3 -> Data Type Conversion2/1  "<red>"
  Bus Selector/4 -> Data Type Conversion3/1  "<green>"
  Bus Selector/5 -> Data Type Conversion4/1  "<blue>"
  flight_mode/1 -> debug8/1, debug7/1, debug6/1, debug5/1, debug4/1, debug3/1, debug1/1
  Data Type Conversion/1 -> led_blue/1
  Data Type Conversion1/1 -> led_red/1
  Data Type Conversion2/1 -> rgb_red/1
  Data Type Conversion3/1 -> rgb_green/1
  Data Type Conversion4/1 -> rgb_blue/1
  Selector11/1 -> debug2/1
  Bus Selector/1 -> Data Type Conversion/1  "<blue_LED>"

== system simulink_app/Status signals ==
  flight_mode : Inport
  Not_allowed_change : Inport  Port=2
  Ground{,1..3} (4 alike) : Ground
  Beep : Outport
  Red_LED : Outport  Port=2
  blue_LED : Outport  Port=3
  blue_RGBLED : Outport  Port=4
  Red_RGBLED : Outport  Port=5
  green_RGBLED : Outport  Port=6
  wires:
  Ground/1 -> blue_RGBLED/1, Red_RGBLED/1, green_RGBLED/1
  Ground1/1 -> Beep/1
  Ground2/1 -> Red_LED/1
  Ground3/1 -> blue_LED/1

== system simulink_app/flight_mode_effector ==
  flight_mode : Inport
  All_meas : Inport  Port=2
  Bus Creator : BusCreator  Inputs=6
  Bus Creator1 : BusCreator  Inputs=6
  Bus Selector1 : BusSelector  OutputSignals=Meas.Pos_meas_m,Params.V_yaw,Meas.Eulr_meas_rad,Meas.omega_b_meas_radps
  alt_act : Memory  X0=false  InheritSampleTime=on
  att_act : Memory  X0=false  InheritSampleTime=on
  flight_mode_effector : MATLAB Function  TreatAsAtomicUnit=on
  man_act : Memory  X0=false  InheritSampleTime=on
  pos_xy_act : Memory  X0=false  InheritSampleTime=on
  vel_yaw_xy_act : Memory  X0=false  InheritSampleTime=on
  vel_yaw_z_act : Memory  X0=false  InheritSampleTime=on
  Act_bus : Outport
  Controller_inits : Outport  Port=2  PortDimensions=12
  CA_reconf : Outport  Port=3
  Armed : Outport  Port=4
  wires:
  flight_mode/1 -> flight_mode_effector/1(flight_mode)
  flight_mode_effector/1(pos_xy_act) -> pos_xy_act/1
  flight_mode_effector/2(alt_act) -> alt_act/1
  flight_mode_effector/3(vel_yaw_xy_act) -> vel_yaw_xy_act/1
  flight_mode_effector/4(vel_yaw_z_act) -> vel_yaw_z_act/1
  flight_mode_effector/5(att_act) -> att_act/1
  flight_mode_effector/6(omega_b_act) -> man_act/1
  flight_mode_effector/9(vel_yaw_xy_init) -> Bus Creator1/3
  flight_mode_effector/12(b_rates_init) -> Bus Creator1/6
  flight_mode_effector/10(vel_yaw_z_init) -> Bus Creator1/4
  flight_mode_effector/11(att_init) -> Bus Creator1/5
  flight_mode_effector/7(pos_xy_init) -> Bus Creator1/1
  flight_mode_effector/8(alt_init) -> Bus Creator1/2
  Bus Selector1/2 -> flight_mode_effector/3(V_yaw)  "<V_yaw>"
  Bus Selector1/1 -> flight_mode_effector/2(X_e)  "<Pos_meas_m>"
  Bus Selector1/3 -> flight_mode_effector/4(Euler)  "<Eulr_meas_rad>"
  Bus Selector1/4 -> flight_mode_effector/5(omega_b)  "<omega_b_meas_radps>"
  pos_xy_act/1 -> Bus Creator/1  "pos_xy_act"
  alt_act/1 -> Bus Creator/2  "alt_act"
  vel_yaw_xy_act/1 -> Bus Creator/3  "vel_yaw_xy_act"
  vel_yaw_z_act/1 -> Bus Creator/4  "vel_yaw_z_act"
  att_act/1 -> Bus Creator/5  "att_act"
  man_act/1 -> Bus Creator/6  "omega_b_act"
  Bus Creator/1 -> Act_bus/1
  Bus Creator1/1 -> Controller_inits/1
  flight_mode_effector/13(CA_reconf) -> CA_reconf/1
  flight_mode_effector/14(Armed) -> Armed/1
  All_meas/1 -> Bus Selector1/1

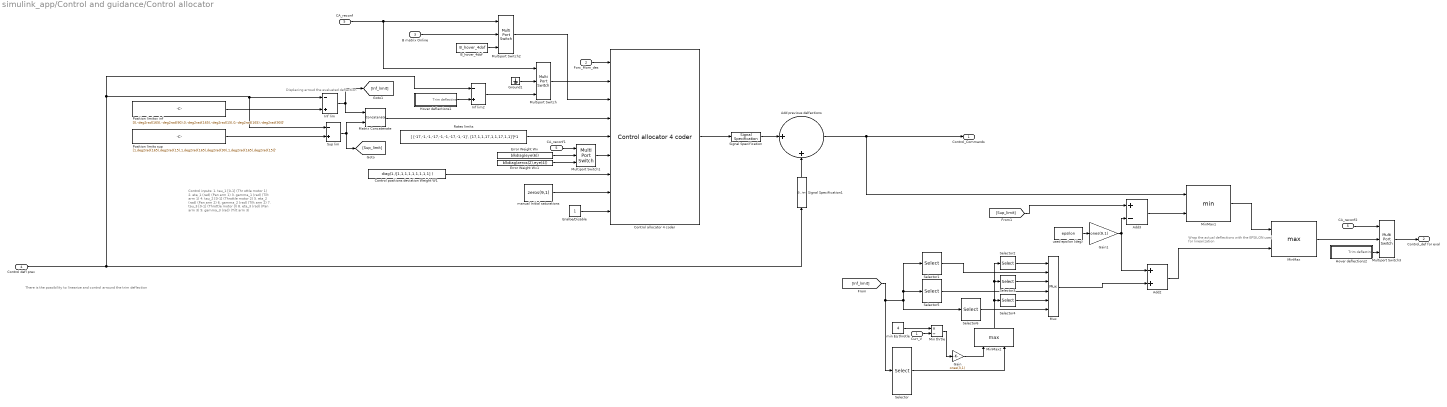
== system simulink_app/Control and guidance/Control allocator ==
  note: There is the possibility to linearize and control arround the trim deflection
  note: Wrap the actual deflections with the EPSILON
      |  used for linearization
  note: Displacing arroud the evaluated deflection
  note: Control inputs:
      | 1. tau_1 [0-1] (Thr ottle motor 1)
      | 2. eta_1 (rad)  (Pan arm 1)
      | 3. gamma_1 (rad)  (Tilt arm 1)
      |
      | 4. tau_2 [0-1] (Throttle motor 2)
      | 5. eta_2 (rad)  (Pan arm 2)
      | 6. gamma_2 (rad)  (Tilt arm 2)
      |
      | 7. tau_3 [0-1] (Throttle motor 3)
      | 8. eta_3 (rad)  (Pan arm  3)
      | 9. gamma_3 (rad)  (Tilt arm 3)
  Curr_V : Inport
  Forc_Mom_des : Inport  Port=2
  B matrix Online : Inport  Port=3
  Control defl prev : Inport  Port=4
  CA_reconf : Inport  Port=5
  Add previous delfections : Sum  Inputs=|++
  Add2 : Sum
  Add3 : Sum  Inputs=+-
  B_hover_4dof : Constant  Value=B_hover_4dof
  CA_reconf1 : InportShadow  Port=5
  CA_reconf2 : InportShadow  Port=5
  Control allocator 4 coder : XXCopter_Control/Control allocator 4 coder  gamma=1  imax=50  T=T_ctrl
  Control positions deviation Weight W1 : Constant  Value=diag(1./[1,1,1,1,1,1,1,1,1] )
  Enalbe/Disable : Constant
  Error Weight Wv : Constant  Value=blkdiag(eye(6))
  Error Weight Wv1 : Constant  Value=blkdiag(zeros(2),eye(4))
  Gain : Gain  Gain=ones(3,1)
  Gain1 : Gain  Gain=ones(9,1)
  Ground1 : Ground
  Hover deflections1 : Subsystem  TreatAsAtomicUnit=on
  Hover deflections2 : Subsystem  TreatAsAtomicUnit=on
  Inf lim : Sum  Inputs=-+
  Inf lim2 : Sum  Inputs=-+
  Matrix Concatenate : Concatenate  Mode=Multidimensional array  ConcatenateDimension=2
  Min thrtle : Product  Inputs=*/
  MinMax : MinMax  Function=max  Inputs=2
  MinMax1 : MinMax  Inputs=2
  MinMax2 : MinMax  Function=max  Inputs=2
  Multiport Switch{,1..3} (4 alike) : MultiPortSwitch  Inputs=2
  Mux : Mux  Inputs=[1,2,1,2,1,2]
  Position limits sup : Constant  Value=[1,deg2rad(165),deg2rad(15),1,deg2rad(165),deg2rad(90),1,deg2rad(165),deg2rad(15)]'
  Position limitsv inf : Constant  Value=[0,-deg2rad(165),-deg2rad(90),0,-deg2rad(165),-deg2rad(15),0,-deg2rad(165),-deg2rad(90)]'
  Rates limits : Constant  Value=[ [-17,-1,-1,-17,-1,-1,-17,-1,-1]', [17,1,1,17,1,1,17,1,1]']*1
  Selector : Selector  InputPortWidth=9  Indices=[1,4,7]
  Selector1 : Selector  InputPortWidth=9  Indices=[2,3]
  Selector2 : Selector  InputPortWidth=3
  Selector3 : Selector  InputPortWidth=3
  Selector4 : Selector  InputPortWidth=3
  Selector5 : Selector  InputPortWidth=9  Indices=[2,3]
  Selector6 : Selector  InputPortWidth=9  Indices=[2,3]
  Signal Specification : SignalSpecification  Dimensions=[9,1]
  Signal Specification1 : SignalSpecification  Dimensions=[9,1]
  Sup lim : Sum  Inputs=-+
  manual Initial saturations : Constant  Value=zeros(9,1)
  min Eq throtle : Constant  Value=4
  used epsilon (deg) : Constant  Value=epsilon
  Control_Commands : Outport
  Control_def for eval : Outport  Port=2
  wires:
  MinMax1/1 -> MinMax/1
  Add3/1 -> MinMax1/2
  used epsilon (deg)/1 -> Gain1/1
  Gain1/1 -> Add2/1, Add3/2
  Add2/1 -> MinMax/2
  Control positions deviation Weight W1/1 -> Control allocator 4 coder/7
  Control allocator 4 coder/1 -> Signal Specification/1
  Enalbe/Disable/1 -> Control allocator 4 coder/9
  manual Initial saturations/1 -> Control allocator 4 coder/8
  Sup lim/1 -> [Sup_limit], Matrix Concatenate/2
  Inf lim/1 -> [Inf_limit], Matrix Concatenate/1
  Position limitsv inf/1 -> Inf lim/2
  Position limits sup/1 -> Sup lim/2
  Rates limits/1 -> Control allocator 4 coder/5
  Add previous delfections/1 -> Control_Commands/1, MinMax1/1
  Multiport Switch2/1 -> Control allocator 4 coder/3
  Signal Specification/1 -> Add previous delfections/1
  Signal Specification1/1 -> Add previous delfections/2
  Forc_Mom_des/1 -> Control allocator 4 coder/1
  Matrix Concatenate/1 -> Control allocator 4 coder/4
  Multiport Switch/1 -> Control allocator 4 coder/2
  Control defl prev/1 -> Signal Specification1/1, Inf lim/1, Sup lim/1, Inf lim2/1
  CA_reconf/1 -> Multiport Switch2/1, Multiport Switch/1
  B matrix Online/1 -> Multiport Switch2/2
  Ground1/1 -> Multiport Switch/2
  Inf lim2/1 -> Multiport Switch/3
  Hover deflections1/1(Trim deflectins) -> Inf lim2/2
  Multiport Switch3/1 -> Control_def for eval/1
  CA_reconf2/1 -> Multiport Switch3/1
  Hover deflections2/1(Trim deflectins) -> Multiport Switch3/3
  MinMax/1 -> Multiport Switch3/2
  B_hover_4dof/1 -> Multiport Switch2/3
  Multiport Switch1/1 -> Control allocator 4 coder/6
  CA_reconf1/1 -> Multiport Switch1/1
  Error Weight Wv/1 -> Multiport Switch1/2
  Error Weight Wv1/1 -> Multiport Switch1/3
  [Inf_limit] -> Selector5/1, Selector1/1, Selector6/1, Selector/1
  Selector/1 -> MinMax2/2
  min Eq throtle/1 -> Min thrtle/1
  Curr_V/1 -> Min thrtle/2
  Min thrtle/1 -> Gain/1
  Gain/1 -> MinMax2/1
  Selector2/1 -> Mux/1
  MinMax2/1 -> Selector4/1, Selector3/1, Selector2/1
  Selector3/1 -> Mux/3
  Selector4/1 -> Mux/5
  Selector1/1 -> Mux/2
  Selector5/1 -> Mux/4
  Selector6/1 -> Mux/6
  Mux/1 -> Add2/2
  [Sup_limit] -> Add3/1

== system simulink_app/Control and guidance/Inner PI Controller Quaternions ==
  Accels ref (m/s^2) : Inport
  Phi_ref (rad) : Inport  Port=2
  Theta_ref (rad) : Inport  Port=3
  Yaw_ref (rad) : Inport  Port=4
  omega_b_ref_radps : Inport  Port=5
  All meas : Inport  Port=6
  activation_bus : Inport  Port=7
  init_cond : Inport  Port=8
  Add : Sum
  Add1 : Sum  Inputs=+-
  Add2 : Sum  Inputs=+-
  All meas1 : InportShadow  Port=6
  Attitude Controller : Subsystem
  Body Rates Controller : Subsystem
  Bus Selector : BusSelector  OutputSignals=Meas.Eulr_meas_rad
  Bus Selector1 : BusSelector  OutputSignals=Meas.q_meas
  Bus Selector2 : BusSelector  OutputSignals=att_act,omega_b_act
  Demux : Demux  Outputs=3
  Get Quaternion from des euler : MATLAB Function  TreatAsAtomicUnit=on
  Limits in Ang accel : Subsystem  TreatAsAtomicUnit=on
  Logical Operator2 : Logic  Operator=NOT  IconShape=distinctive  AllPortsSameDT=off  OutDataTypeStr=boolean
  Logical Operator3 : Logic  IconShape=distinctive  AllPortsSameDT=off  OutDataTypeStr=boolean
  MATLAB Function : MATLAB Function  TreatAsAtomicUnit=on
  Memory : Memory  X0=[0;0;0]  InheritSampleTime=on
  Mux : Mux  Inputs=2
  Quaternion_dot : MATLAB Function  TreatAsAtomicUnit=on  VariantControl=Variant
  Saturation1 : Saturate  UpperLimit=deg2rad(50)*[1,10,0.5]'  LowerLimit=-deg2rad(50)*[1,10,0.5]'
  Switch1 : Switch  Criteria=u2 ~= 0
  T : Gain  Gain=T_ctrl
  Accs_Ang_acc des : Outport
  wires:
  Accels ref (m/s^2)/1 -> Mux/1
  Mux/1 -> Accs_Ang_acc des/1
  All meas/1 -> Bus Selector/1, Attitude Controller/5(All_meas)
  Bus Selector/1 -> Limits in Ang accel/2(Euler meas), MATLAB Function/2(Euler)  "<Eulr_meas_rad>"
  Demux/1 -> Body Rates Controller/1(p_ref)
  Demux/2 -> Body Rates Controller/2(q_ref)
  Demux/3 -> Body Rates Controller/3(r_ref)
  Phi_ref (rad)/1 -> Attitude Controller/2(Phi_ref (rad)), Get Quaternion from des euler/1(phi)
  Theta_ref (rad)/1 -> Get Quaternion from des euler/2(theta)
  Yaw_ref (rad)/1 -> Attitude Controller/4(Yaw_ref (rad)), Get Quaternion from des euler/3(psi)
  Bus Selector1/1 -> Quaternion_dot/2(q)  "<q_meas>"
  Get Quaternion from des euler/1(q) -> Attitude Controller/3(q_ref)
  Attitude Controller/1(quat_dot des (rad/s)) -> Quaternion_dot/1(q_dot)
  Limits in Ang accel/1(ang Ace des) -> Add2/1, Mux/2
  Switch1/1 -> Add1/2, Saturation1/1
  Body Rates Controller/1(Angular acc des (rad/s^2)) -> Add2/2, Limits in Ang accel/1(Ang Ace des)
  Add/1 -> MATLAB Function/1(omega_b)
  Add2/1 -> T/1
  Add1/1 -> Add/2
  T/1 -> Add/1
  MATLAB Function/1(Euler_dot) -> Memory/1
  init_cond/1 -> Body Rates Controller/5(init_cond), Attitude Controller/7(init_cond)
  activation_bus/1 -> Attitude Controller/6(activation_bus), Bus Selector2/1, Body Rates Controller/6(activation_bus)
  All meas1/1 -> Body Rates Controller/4(All_meas), Bus Selector1/1
  Bus Selector2/1 -> Logical Operator2/1  "<att_act>"
  Logical Operator2/1 -> Logical Operator3/1
  Bus Selector2/2 -> Logical Operator3/2  "<omega_b_act>"
  Saturation1/1 -> Demux/1, Add1/1
  Logical Operator3/1 -> Switch1/2
  Quaternion_dot/1(omega_b) -> Switch1/3
  omega_b_ref_radps/1 -> Switch1/1
  Memory/1 -> Attitude Controller/1(AWU)

== system simulink_app/Control and guidance/NDI ==
  note: Rejection for the
      | angular accelerations
  note: Pseudo control inputs:
      | 1. Desired angular accelerations (rad/s^2)
      | 2. Desired accelerations (m/s^2) in body axes
  pseudo_control (m/s^2;rad/s^2) : Inport
  Control_defl for eval : Inport  Port=2
  All_meas : Inport  Port=3
  3Copter_4_NDI&CA : Subsystem  TreatAsAtomicUnit=on
  Bus Selector : BusSelector  OutputSignals=Meas.omega_b_meas_radps,Meas.q_meas,Meas.V_b_meas,Meas.Alt_meas_m,Meas.Volt
  Demux : Demux  Outputs=[3,3]
  Derivative1 : Derivative  CoefficientInTFapproximation=500
  Ground : Ground
  Ground1 : Ground
  Inversion : Sum  Inputs=|+-
  Mux : Mux  Inputs=[3,3]
  Mux2 : Mux  Inputs=[3,3]
  Rot eqs_ Get moments : XXCopter_Control/Rot eqs_ Get moments
  Transl Eqs_ Get forces : XXCopter_Control/Transl Eqs_ Get forces
  "angles " : Selector  IndexMode=Zero-based  InputPortWidth=9  Indices=[1,2,4,5,7,8]
  epsilon (rad or unitary) : Constant  Value=epsilon
  m : Constant  Value=m
  m1 : Constant  Value=m
  Virtual Control Commands : Outport
  B online : Outport  Port=2
  Control_defl eval (rad) : Outport  Port=3
  wires:
  3Copter_4_NDI&CA/3(CA_grad) -> B online/1
  Mux/1 -> Inversion/1
  Mux2/1 -> Inversion/2  "f_x(x)"
  All_meas/1 -> Bus Selector/1
  pseudo_control (m/s^2;rad/s^2)/1 -> Demux/1
  Demux/2 -> Rot eqs_ Get moments/2, Transl Eqs_ Get forces/4
  Demux/1 -> Transl Eqs_ Get forces/1
  Bus Selector/1 -> Transl Eqs_ Get forces/3, Rot eqs_ Get moments/1, 3Copter_4_NDI&CA/6(omega_b)  "<omega_b_meas_radps>"
  Bus Selector/3 -> Transl Eqs_ Get forces/2, 3Copter_4_NDI&CA/4(Vb)  "<V_b_meas>"
  3Copter_4_NDI&CA/4(I_BAC) -> Rot eqs_ Get moments/3
  3Copter_4_NDI&CA/5("CG ") -> Transl Eqs_ Get forces/6
  Control_defl for eval/1 -> 3Copter_4_NDI&CA/2(Control Inputs (rad)), Control_defl eval (rad)/1, "angles "/1
  Bus Selector/4 -> 3Copter_4_NDI&CA/3(h)  "<Alt_meas_m>"
  Bus Selector/2 -> 3Copter_4_NDI&CA/5(q)  "<q_meas>"
  m1/1 -> 3Copter_4_NDI&CA/11(" m")
  m/1 -> Transl Eqs_ Get forces/5
  epsilon (rad or unitary)/1 -> 3Copter_4_NDI&CA/1("epsilon (rad or unitary) ")
  Transl Eqs_ Get forces/1 -> Mux/1
  Rot eqs_ Get moments/1 -> Mux/2
  3Copter_4_NDI&CA/1(Forces) -> Mux2/1
  3Copter_4_NDI&CA/2(Moments) -> Mux2/2
  Inversion/1 -> Virtual Control Commands/1
  Ground/1 -> 3Copter_4_NDI&CA/7(Omegas_dot_actual)
  "angles "/1 -> Derivative1/1, 3Copter_4_NDI&CA/8(angles_actual)
  Derivative1/1 -> 3Copter_4_NDI&CA/9(angles_dot_actual)
  Ground1/1 -> 3Copter_4_NDI&CA/10(angles_dot_dot_actual)
  Bus Selector/5 -> 3Copter_4_NDI&CA/12(Curr_V)  "<Volt>"
